simulink model "nmsRR"  (R2021a)
settings: Solver=ode15s  StartTime=0.0  StopTime=t  MaxStep=1e-2  RelTol=1e-2
StartFcn:
  | tic
StopFcn:
  | toc
  | 
  | 
  | %if GimbalLockFlag
  |  % fprintf(2, 'Almost reached Gimbal Lock of IMU. Simulation stopped.\n')
  | %end
  | 
  | %fprintf('Elapsed time: %4.2f sec (%4.2f%% realtime)\n', a, tout(end)/a*100)
undefined symbols (not defined in the file): Balance02, Balance13, BalanceTrunk, BasisStim, CompensateSwing, CompliantLeg, FlexAnkle, Ground, ICs, init_des_left, init_des_right, init_l_left, init_l_right, init_q_del, init_sensor_body, init_sensor_world, init_v_left, init_v_right, LateralControl, mParams, PreventKneeOverextension, StepDur, Target02, Target13, theta0, X, Y, Z
libraries: simulink_extras x133, nesl_utility x105, sm_lib x88, simulink x72, robotcorelib x5, dspinverses x5, dspswit3 x2, vrlib x2, robotmaniplib x1
(part 2 of 8)

== system nmsRR/Body and Contact Model/LPF 13x0.01s3 ==
  in : Inport
  Demux2 : Demux  Outputs=8
  Mux2 : Mux  Inputs=8
  Transfer Fcn (with initial outputs){,1..7} (8 alike) : simulink_extras/Additional Linear/Transfer Fcn (with initial outputs)  N=[1]  D="[0.01  1]"  Y0=0  U0=0
  Out : Outport
  wires:
  Mux2/1 -> Out/1
  in/1 -> Demux2/1
  Demux2/1 -> Transfer Fcn (with initial outputs)/1
  Transfer Fcn (with initial outputs)/1 -> Mux2/1
  Demux2/2 -> Transfer Fcn (with initial outputs)1/1
  Transfer Fcn (with initial outputs)1/1 -> Mux2/2
  Demux2/3 -> Transfer Fcn (with initial outputs)2/1
  Transfer Fcn (with initial outputs)2/1 -> Mux2/3
  Demux2/4 -> Transfer Fcn (with initial outputs)3/1
  Transfer Fcn (with initial outputs)3/1 -> Mux2/4
  Demux2/5 -> Transfer Fcn (with initial outputs)4/1
  Transfer Fcn (with initial outputs)4/1 -> Mux2/5
  Demux2/6 -> Transfer Fcn (with initial outputs)5/1
  Transfer Fcn (with initial outputs)5/1 -> Mux2/6
  Demux2/7 -> Transfer Fcn (with initial outputs)6/1
  Transfer Fcn (with initial outputs)6/1 -> Mux2/7
  Demux2/8 -> Transfer Fcn (with initial outputs)7/1
  Transfer Fcn (with initial outputs)7/1 -> Mux2/8

== system nmsRR/Body and Contact Model/LPF 13x0.01s4 ==
  in : Inport
  Demux2 : Demux  Outputs=8
  Mux2 : Mux  Inputs=8
  Transfer Fcn (with initial outputs) : simulink_extras/Additional Linear/Transfer Fcn (with initial outputs)  N=[1]  D="[0.01  1]"  Y0=init_q_del(1)  U0=init_q_del(1)
  Transfer Fcn (with initial outputs)1 : simulink_extras/Additional Linear/Transfer Fcn (with initial outputs)  N=[1]  D="[0.01  1]"  Y0=init_q_del(2)  U0=init_q_del(2)
  Transfer Fcn (with initial outputs)2 : simulink_extras/Additional Linear/Transfer Fcn (with initial outputs)  N=[1]  D="[0.01  1]"  Y0=init_q_del(3)  U0=init_q_del(3)
  Transfer Fcn (with initial outputs)3 : simulink_extras/Additional Linear/Transfer Fcn (with initial outputs)  N=[1]  D="[0.01  1]"  Y0=init_q_del(4)  U0=init_q_del(4)
  Transfer Fcn (with initial outputs)4 : simulink_extras/Additional Linear/Transfer Fcn (with initial outputs)  N=[1]  D="[0.01  1]"  Y0=init_q_del(5)  U0=init_q_del(5)
  Transfer Fcn (with initial outputs)5 : simulink_extras/Additional Linear/Transfer Fcn (with initial outputs)  N=[1]  D="[0.01  1]"  Y0=init_q_del(6)  U0=init_q_del(6)
  Transfer Fcn (with initial outputs)6 : simulink_extras/Additional Linear/Transfer Fcn (with initial outputs)  N=[1]  D="[0.01  1]"  Y0=0  U0=0
  Transfer Fcn (with initial outputs)7 : simulink_extras/Additional Linear/Transfer Fcn (with initial outputs)  N=[1]  D="[0.01  1]"  Y0=0  U0=0
  Out : Outport
  wires:
  Mux2/1 -> Out/1
  in/1 -> Demux2/1
  Demux2/1 -> Transfer Fcn (with initial outputs)/1
  Transfer Fcn (with initial outputs)/1 -> Mux2/1
  Demux2/2 -> Transfer Fcn (with initial outputs)1/1
  Transfer Fcn (with initial outputs)1/1 -> Mux2/2
  Demux2/3 -> Transfer Fcn (with initial outputs)2/1
  Transfer Fcn (with initial outputs)2/1 -> Mux2/3
  Demux2/4 -> Transfer Fcn (with initial outputs)3/1
  Transfer Fcn (with initial outputs)3/1 -> Mux2/4
  Demux2/5 -> Transfer Fcn (with initial outputs)4/1
  Transfer Fcn (with initial outputs)4/1 -> Mux2/5
  Demux2/6 -> Transfer Fcn (with initial outputs)5/1
  Transfer Fcn (with initial outputs)5/1 -> Mux2/6
  Demux2/7 -> Transfer Fcn (with initial outputs)6/1
  Transfer Fcn (with initial outputs)6/1 -> Mux2/7
  Demux2/8 -> Transfer Fcn (with initial outputs)7/1
  Transfer Fcn (with initial outputs)7/1 -> Mux2/8

== system nmsRR/Body and Contact Model/Push in x-direction ==
  Left/Right : Inport
  " Timer Phase 1" : Subsystem
  AND : Logic  AllPortsSameDT=off  OutDataTypeStr=boolean
  Compare To Constant : simulink/Logic and Bit Operations/Compare To Constant  relop===  const=10  OutDataTypeStr=boolean  ZeroCross=off
  Compare To Constant1 : simulink/Logic and Bit Operations/Compare To Constant  relop=<=  const=0.2  OutDataTypeStr=boolean
  Constant1 : Constant  Value=-135
  Constant3 : Constant  Value=0
  Counter : dspswit3/Counter  Direction=Up  CountEvent=Rising edge  CounterSize=User defined  MaxCount=255  InitialCount=0  Output=Count and Hit  HitValue=32  ResetInput=off  SamplesPerFrame=1  Ts=1  CntDtype=double  HitDtype=Logical
  External Force and Torque : sm_lib/Forces and Torques/External Force and Torque  ForceResolutionFrame=AttachedFrame  EnableForceX=on  EnableForceY=off  EnableForceZ=off  EnableForce=off  TorqueResolutionFrame=AttachedFrame  EnableTorqueX=off  EnableTorqueY=off  EnableTorqueZ=off  EnableTorque=off
  Switch : Switch  Criteria=u2 > Threshold
  Terminator2 : Terminator
  conversion : nesl_utility/Simulink-PS Converter  PhysicalDomain=network_engine_domain  SubClassName=ps_input  LeftPortType=input  RightPortType=output  PseudoPeriodic=off  Frequencies=[]  NoiseDistribution=none  NoiseParameters=[]  Unit=N  AffineConversion=off  FilteringAndDerivatives=zero  SimscapeFilterOrder=1  InputFilterTimeConstant=.001  UdotUserProvided=0
      settings: SourceProductBaseCode=PW,SS
  External Force [100 N] : PMIOPort  Side=Right
  wires:
  " Timer Phase 1"/1(Out) -> Compare To Constant1/1
  Compare To Constant/1 -> AND/1, " Timer Phase 1"/1(R)
  Counter/2 -> Terminator2/1
  Compare To Constant1/1 -> AND/2
  Left/Right/1 -> Counter/1
  Constant3/1 -> Switch/3
  AND/1 -> Switch/2
  Switch/1 -> conversion/1
  Constant1/1 -> Switch/1
  Counter/1 -> Compare To Constant/1
  connections:
  conversion/RConn1 -- External Force and Torque/LConn1
  External Force and Torque/RConn1 -- External Force [100 N]/RConn1

== system nmsRR/Body and Contact Model/Push in y-direction ==
  Left/Right : Inport
  " Timer Phase 1" : Subsystem
  AND : Logic  AllPortsSameDT=off  OutDataTypeStr=boolean
  Compare To Constant : simulink/Logic and Bit Operations/Compare To Constant  relop===  const=10  OutDataTypeStr=boolean  ZeroCross=off
  Compare To Constant1 : simulink/Logic and Bit Operations/Compare To Constant  relop=<=  const=0.2  OutDataTypeStr=boolean
  Constant1 : Constant  Value=-360
  Constant3 : Constant  Value=0
  Counter : dspswit3/Counter  Direction=Up  CountEvent=Rising edge  CounterSize=User defined  MaxCount=255  InitialCount=0  Output=Count and Hit  HitValue=32  ResetInput=off  SamplesPerFrame=1  Ts=1  CntDtype=double  HitDtype=Logical
  External Force and Torque : sm_lib/Forces and Torques/External Force and Torque  ForceResolutionFrame=AttachedFrame  EnableForceX=off  EnableForceY=off  EnableForceZ=on  EnableForce=off  TorqueResolutionFrame=AttachedFrame  EnableTorqueX=off  EnableTorqueY=off  EnableTorqueZ=off  EnableTorque=off
  Switch : Switch  Criteria=u2 > Threshold
  Terminator2 : Terminator
  conversion : nesl_utility/Simulink-PS Converter  PhysicalDomain=network_engine_domain  SubClassName=ps_input  LeftPortType=input  RightPortType=output  PseudoPeriodic=off  Frequencies=[]  NoiseDistribution=none  NoiseParameters=[]  Unit=N  AffineConversion=off  FilteringAndDerivatives=zero  SimscapeFilterOrder=1  InputFilterTimeConstant=.001  UdotUserProvided=0
      settings: SourceProductBaseCode=PW,SS
  External Force [100 N] : PMIOPort  Side=Right
  wires:
  " Timer Phase 1"/1(Out) -> Compare To Constant1/1
  Compare To Constant/1 -> AND/1, " Timer Phase 1"/1(R)
  Counter/2 -> Terminator2/1
  Compare To Constant1/1 -> AND/2
  Left/Right/1 -> Counter/1
  Constant3/1 -> Switch/3
  AND/1 -> Switch/2
  Switch/1 -> conversion/1
  Constant1/1 -> Switch/1
  Counter/1 -> Compare To Constant/1
  connections:
  conversion/RConn1 -- External Force and Torque/LConn1
  External Force and Torque/RConn1 -- External Force [100 N]/RConn1

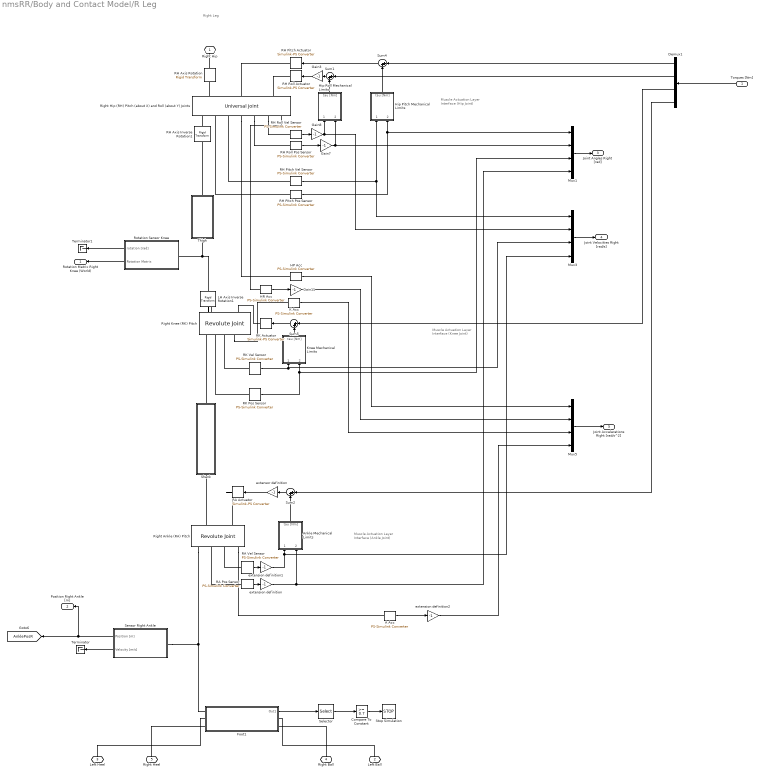
== system nmsRR/Body and Contact Model/R Leg ==
  note: Muscle Actuation
      | Layer Interface
      | (Hip Joint)
  note: Muscle Actuation
      | Layer Interface
      | (Knee Joint)
  note: Muscle Actuation
      | Layer Interface
      | (Ankle Joint)
  note: Right Leg
  Torques [Nm] : Inport
  A Acc : nesl_utility/PS-Simulink Converter  PhysicalDomain=network_engine_domain  SubClassName=ps_output  LeftPortType=input  RightPortType=output  PseudoPeriodic=off  Frequencies=[]  Unit=rad/(s^2)  AffineConversion=off
      settings: SourceProductBaseCode=PW,SS
  Ankle Mechanical Limits : Subsystem
  Compare To Constant : simulink/Logic and Bit Operations/Compare To Constant  relop=>=  const=0.7  OutDataTypeStr=boolean
  Demux1 : Demux
  Foot1 : Subsystem
  Gain{3,7..8,11} (4 alike) : Gain  Gain=-1
  HP Acc : nesl_utility/PS-Simulink Converter  PhysicalDomain=network_engine_domain  SubClassName=ps_output  LeftPortType=input  RightPortType=output  PseudoPeriodic=off  Frequencies=[]  Unit=rad/(s^2)  AffineConversion=off
      settings: SourceProductBaseCode=PW,SS
  HR Acc : nesl_utility/PS-Simulink Converter  PhysicalDomain=network_engine_domain  SubClassName=ps_output  LeftPortType=input  RightPortType=output  PseudoPeriodic=off  Frequencies=[]  Unit=rad/(s^2)  AffineConversion=off
      settings: SourceProductBaseCode=PW,SS
  Hip Pitch Mechanical Limits : Subsystem
  Hip Roll Mechanical Limits : Subsystem
  K Acc : nesl_utility/PS-Simulink Converter  PhysicalDomain=network_engine_domain  SubClassName=ps_output  LeftPortType=input  RightPortType=output  PseudoPeriodic=off  Frequencies=[]  Unit=rad/(s^2)  AffineConversion=off
      settings: SourceProductBaseCode=PW,SS
  Knee Mechanical Limits : Subsystem
  LH Axis Inverse Rotation1 : sm_lib/Frames and Transforms/Rigid Transform  TranslationMethod=None  TranslationStandardOffset=-0.5  TranslationLengthUnit=m  TranslationStandardAxis=+Y  TranslationCartesianOffset=0  TranslationROffset=0  TranslationROffsetUnits=m  TranslationZOffset=0  TranslationZOffsetUnits=m  TranslationThetaOffset=0  TranslationThetaOffsetUnits=deg  RotationMethod=RotationSequence  RotationAngleUnits=deg  RotationStandardAxis=+X  RotationAngle=-90  RotationArbitraryAxis=[0 0 1]  FollAlignAxisA=+X  BaseAlignAxisA=+Y  FollAlignAxisB=+Y  BaseAlignAxisB=+Z  RotationSequenceAxes=BaseAxes  RotationSequence=ZXZ  RotationSequenceAngles=[180 0 0]  RotationSequenceAnglesUnits=deg  RotationMatrix=[1 0 0; 0 1 0; 0 0 1]
  Mux1 : Mux
  Mux3 : Mux
  Mux5 : Mux
  RA Actuator : nesl_utility/Simulink-PS Converter  PhysicalDomain=network_engine_domain  SubClassName=ps_input  LeftPortType=input  RightPortType=output  PseudoPeriodic=off  Frequencies=[]  NoiseDistribution=none  NoiseParameters=[]  Unit=N*m  AffineConversion=off  FilteringAndDerivatives=zero  SimscapeFilterOrder=1  InputFilterTimeConstant=.001  UdotUserProvided=0
      settings: SourceProductBaseCode=PW,SS
  RA Pos Sensor : nesl_utility/PS-Simulink Converter  PhysicalDomain=network_engine_domain  SubClassName=ps_output  LeftPortType=input  RightPortType=output  PseudoPeriodic=off  Frequencies=[]  Unit=rad  AffineConversion=off
      settings: SourceProductBaseCode=PW,SS
  RA Vel Sensor : nesl_utility/PS-Simulink Converter  PhysicalDomain=network_engine_domain  SubClassName=ps_output  LeftPortType=input  RightPortType=output  PseudoPeriodic=off  Frequencies=[]  Unit=rad/s  AffineConversion=off
      settings: SourceProductBaseCode=PW,SS
  RH Pitch Pos Sensor : nesl_utility/PS-Simulink Converter  PhysicalDomain=network_engine_domain  SubClassName=ps_output  LeftPortType=input  RightPortType=output  PseudoPeriodic=off  Frequencies=[]  Unit=rad  AffineConversion=off
      settings: SourceProductBaseCode=PW,SS
  RH Pitch Vel Sensor : nesl_utility/PS-Simulink Converter  PhysicalDomain=network_engine_domain  SubClassName=ps_output  LeftPortType=input  RightPortType=output  PseudoPeriodic=off  Frequencies=[]  Unit=rad/s  AffineConversion=off
      settings: SourceProductBaseCode=PW,SS
  RH Roll Pos Sensor : nesl_utility/PS-Simulink Converter  PhysicalDomain=network_engine_domain  SubClassName=ps_output  LeftPortType=input  RightPortType=output  PseudoPeriodic=off  Frequencies=[]  Unit=rad  AffineConversion=off
      settings: SourceProductBaseCode=PW,SS
  "RH Roll Vel Sensor " : nesl_utility/PS-Simulink Converter  PhysicalDomain=network_engine_domain  SubClassName=ps_output  LeftPortType=input  RightPortType=output  PseudoPeriodic=off  Frequencies=[]  Unit=rad/s  AffineConversion=off
      settings: SourceProductBaseCode=PW,SS
  RH Axis Inverse Rotation1 : sm_lib/Frames and Transforms/Rigid Transform  TranslationMethod=None  TranslationStandardOffset=-0.5  TranslationLengthUnit=m  TranslationStandardAxis=+Y  TranslationCartesianOffset=[0 0.2 0]  TranslationROffset=0  TranslationROffsetUnits=m  TranslationZOffset=0  TranslationZOffsetUnits=m  TranslationThetaOffset=0  TranslationThetaOffsetUnits=deg  RotationMethod=RotationSequence  RotationAngleUnits=deg  RotationStandardAxis=+X  RotationAngle=-90  RotationArbitraryAxis=[0 0 1]  FollAlignAxisA=+X  BaseAlignAxisA=+Y  FollAlignAxisB=+Y  BaseAlignAxisB=+Z  RotationSequenceAxes=BaseAxes  RotationSequence=YXY  RotationSequenceAngles=[ -90 -90 0]  RotationSequenceAnglesUnits=deg  RotationMatrix=[1 0 0; 0 1 0; 0 0 1]
  RH Axis Rotation : sm_lib/Frames and Transforms/Rigid Transform  TranslationMethod=None  TranslationStandardOffset=-0  TranslationLengthUnit=m  TranslationStandardAxis=+Y  TranslationCartesianOffset=0  TranslationROffset=0  TranslationROffsetUnits=m  TranslationZOffset=0  TranslationZOffsetUnits=m  TranslationThetaOffset=0  TranslationThetaOffsetUnits=deg  RotationMethod=RotationSequence  RotationAngleUnits=deg  RotationStandardAxis=+X  RotationAngle=90  RotationArbitraryAxis=[0 0 1]  FollAlignAxisA=+X  BaseAlignAxisA=+Y  FollAlignAxisB=+Y  BaseAlignAxisB=+Z  RotationSequenceAxes=FollowerAxes  RotationSequence=XZX  RotationSequenceAngles=[-90 90 0]  RotationSequenceAnglesUnits=deg  RotationMatrix=[1 0 0; 0 1 0; 0 0 1]
  RH Pitch Actuator : nesl_utility/Simulink-PS Converter  PhysicalDomain=network_engine_domain  SubClassName=ps_input  LeftPortType=input  RightPortType=output  PseudoPeriodic=off  Frequencies=[]  NoiseDistribution=none  NoiseParameters=[]  Unit=N*m  AffineConversion=off  FilteringAndDerivatives=zero  SimscapeFilterOrder=1  InputFilterTimeConstant=.001  UdotUserProvided=0
      settings: SourceProductBaseCode=PW,SS
  RH Roll Actuator : nesl_utility/Simulink-PS Converter  PhysicalDomain=network_engine_domain  SubClassName=ps_input  LeftPortType=input  RightPortType=output  PseudoPeriodic=off  Frequencies=[]  NoiseDistribution=none  NoiseParameters=[]  Unit=N*m  AffineConversion=off  FilteringAndDerivatives=zero  SimscapeFilterOrder=1  InputFilterTimeConstant=.001  UdotUserProvided=0
      settings: SourceProductBaseCode=PW,SS
  RK Actuator : nesl_utility/Simulink-PS Converter  PhysicalDomain=network_engine_domain  SubClassName=ps_input  LeftPortType=input  RightPortType=output  PseudoPeriodic=off  Frequencies=[]  NoiseDistribution=none  NoiseParameters=[]  Unit=N*m  AffineConversion=off  FilteringAndDerivatives=zero  SimscapeFilterOrder=1  InputFilterTimeConstant=.001  UdotUserProvided=0
      settings: SourceProductBaseCode=PW,SS
  RK Pos Sensor : nesl_utility/PS-Simulink Converter  PhysicalDomain=network_engine_domain  SubClassName=ps_output  LeftPortType=input  RightPortType=output  PseudoPeriodic=off  Frequencies=[]  Unit=rad  AffineConversion=off
      settings: SourceProductBaseCode=PW,SS
  RK Vel Sensor : nesl_utility/PS-Simulink Converter  PhysicalDomain=network_engine_domain  SubClassName=ps_output  LeftPortType=input  RightPortType=output  PseudoPeriodic=off  Frequencies=[]  Unit=rad/s  AffineConversion=off
      settings: SourceProductBaseCode=PW,SS
  Right Ankle (RA) Pitch : sm_lib/Joints/Revolute Joint  JointMode=Normal  SenseConstraintForce=off  SenseConstraintForceX=off  SenseConstraintForceY=off  SenseConstraintForceZ=off  SenseConstraintTorque=off  SenseConstraintTorqueX=off  SenseConstraintTorqueY=off  SenseConstraintTorqueZ=off  SenseTotalForce=off  SenseTotalForceX=off  SenseTotalForceY=off  SenseTotalForceZ=off  SenseTotalTorque=off  SenseTotalTorqueX=off  SenseTotalTorqueY=off  SenseTotalTorqueZ=off  CompositeWrenchDir=FollowerOnBase  CompositeWrenchFrame=FollowerFrame  EquilibriumPosition=0  EquilibriumPositionUnits=deg  SpringStiffness=0  SpringStiffnessUnits=N*m/deg  DampingCoefficient=0  DampingCoefficientUnits=N*m/(deg/s)  TorqueActuationMode=InputTorque  MotionActuationMode=ComputedMotion  SensePosition=on  SenseVelocity=on  SenseAcceleration=on  SenseTorqueForce=off  SenseLowerLimitTorqueForce=off  SenseUpperLimitTorqueForce=off  LowerLimitSpecify=off  LowerLimitBound=-90  LowerLimitBoundUnits=deg  LowerLimitStiffness=1e4  LowerLimitStiffnessUnits=N*m/deg  LowerLimitDamping=10  LowerLimitDampingUnits=N*m/(deg/s)  LowerLimitTransitionRegionWidth=0.1  LowerLimitTransitionRegionWidthUnits=deg  UpperLimitSpecify=off  UpperLimitBound=90  UpperLimitBoundUnits=deg  UpperLimitStiffness=1e4  UpperLimitStiffnessUnits=N*m/deg  UpperLimitDamping=10  UpperLimitDampingUnits=N*m/(deg/s)  UpperLimitTransitionRegionWidth=0.1  UpperLimitTransitionRegionWidthUnits=deg  PositionTargetSpecify=on  PositionTargetPriority=High  PositionTargetValue=-ICs.rLeg.ankle.qP0  PositionTargetValueUnits=rad  VelocityTargetSpecify=on  VelocityTargetPriority=High  VelocityTargetValue=0  VelocityTargetValueUnits=rad/s
  Right Hip (RH) Pitch (about X) and Roll (about Y) Joints : sm_lib/Joints/Universal Joint  JointMode=Normal  SenseConstraintForce=off  SenseConstraintForceX=off  SenseConstraintForceY=off  SenseConstraintForceZ=off  SenseConstraintTorque=off  SenseConstraintTorqueX=off  SenseConstraintTorqueY=off  SenseConstraintTorqueZ=off  SenseTotalForce=off  SenseTotalForceX=off  SenseTotalForceY=off  SenseTotalForceZ=off  SenseTotalTorque=off  SenseTotalTorqueX=off  SenseTotalTorqueY=off  SenseTotalTorqueZ=off  CompositeWrenchDir=FollowerOnBase  CompositeWrenchFrame=FollowerFrame  RxEquilibriumPosition=0  RxEquilibriumPositionUnits=deg  RxSpringStiffness=0  RxSpringStiffnessUnits=N*m/deg  RxDampingCoefficient=0  RxDampingCoefficientUnits=N*m/(deg/s)  RxTorqueActuationMode=InputTorque  RxMotionActuationMode=ComputedMotion  RxSensePosition=on  RxSenseVelocity=on  RxSenseAcceleration=on  RxSenseTorqueForce=off  RxSenseLowerLimitTorqueForce=off  RxSenseUpperLimitTorqueForce=off  RxLowerLimitSpecify=off  RxLowerLimitBound=-90  RxLowerLimitBoundUnits=deg  RxLowerLimitStiffness=1e4  RxLowerLimitStiffnessUnits=N*m/deg  RxLowerLimitDamping=10  RxLowerLimitDampingUnits=N*m/(deg/s)  RxLowerLimitTransitionRegionWidth=0.1  RxLowerLimitTransitionRegionWidthUnits=deg  RxUpperLimitSpecify=off  RxUpperLimitBound=90  RxUpperLimitBoundUnits=deg  RxUpperLimitStiffness=1e4  RxUpperLimitStiffnessUnits=N*m/deg  RxUpperLimitDamping=10  RxUpperLimitDampingUnits=N*m/(deg/s)  RxUpperLimitTransitionRegionWidth=0.1  RxUpperLimitTransitionRegionWidthUnits=deg  RxPositionTargetSpecify=on  RxPositionTargetPriority=High  RxPositionTargetValue=ICs.rLeg.hip.qP0  RxPositionTargetValueUnits=rad  RxVelocityTargetSpecify=on  RxVelocityTargetPriority=High  RxVelocityTargetValue=0  RxVelocityTargetValueUnits=rad/s  RyEquilibriumPosition=0  RyEquilibriumPositionUnits=deg  RySpringStiffness=0  RySpringStiffnessUnits=N*m/deg  RyDampingCoefficient=0  RyDampingCoefficientUnits=N*m/(deg/s)  RyTorqueActuationMode=InputTorque  RyMotionActuationMode=ComputedMotion  RySensePosition=on  RySenseVelocity=on  RySenseAcceleration=on  RySenseTorqueForce=off  RySenseLowerLimitTorqueForce=off  RySenseUpperLimitTorqueForce=off  RyLowerLimitSpecify=off  RyLowerLimitBound=-90  RyLowerLimitBoundUnits=deg  RyLowerLimitStiffness=1e4  RyLowerLimitStiffnessUnits=N*m/deg  RyLowerLimitDamping=10  RyLowerLimitDampingUnits=N*m/(deg/s)  RyLowerLimitTransitionRegionWidth=0.1  RyLowerLimitTransitionRegionWidthUnits=deg  RyUpperLimitSpecify=off  RyUpperLimitBound=90  RyUpperLimitBoundUnits=deg  RyUpperLimitStiffness=1e4  RyUpperLimitStiffnessUnits=N*m/deg  RyUpperLimitDamping=10  RyUpperLimitDampingUnits=N*m/(deg/s)  RyUpperLimitTransitionRegionWidth=0.1  RyUpperLimitTransitionRegionWidthUnits=deg  RyPositionTargetSpecify=on  RyPositionTargetPriority=High  RyPositionTargetValue=-ICs.rLeg.hip.qR0  RyPositionTargetValueUnits=rad  RyVelocityTargetSpecify=on  RyVelocityTargetPriority=High  RyVelocityTargetValue=0  RyVelocityTargetValueUnits=rad/s
  Right Knee (RK) Pitch : sm_lib/Joints/Revolute Joint  JointMode=Normal  SenseConstraintForce=off  SenseConstraintForceX=off  SenseConstraintForceY=off  SenseConstraintForceZ=off  SenseConstraintTorque=off  SenseConstraintTorqueX=off  SenseConstraintTorqueY=off  SenseConstraintTorqueZ=off  SenseTotalForce=off  SenseTotalForceX=off  SenseTotalForceY=off  SenseTotalForceZ=off  SenseTotalTorque=off  SenseTotalTorqueX=off  SenseTotalTorqueY=off  SenseTotalTorqueZ=off  CompositeWrenchDir=FollowerOnBase  CompositeWrenchFrame=FollowerFrame  EquilibriumPosition=0  EquilibriumPositionUnits=deg  SpringStiffness=0  SpringStiffnessUnits=N*m/deg  DampingCoefficient=0  DampingCoefficientUnits=N*m/(deg/s)  TorqueActuationMode=InputTorque  MotionActuationMode=ComputedMotion  SensePosition=on  SenseVelocity=on  SenseAcceleration=on  SenseTorqueForce=on  SenseLowerLimitTorqueForce=off  SenseUpperLimitTorqueForce=off  LowerLimitSpecify=off  LowerLimitBound=-90  LowerLimitBoundUnits=deg  LowerLimitStiffness=1e4  LowerLimitStiffnessUnits=N*m/deg  LowerLimitDamping=10  LowerLimitDampingUnits=N*m/(deg/s)  LowerLimitTransitionRegionWidth=0.1  LowerLimitTransitionRegionWidthUnits=deg  UpperLimitSpecify=off  UpperLimitBound=90  UpperLimitBoundUnits=deg  UpperLimitStiffness=1e4  UpperLimitStiffnessUnits=N*m/deg  UpperLimitDamping=10  UpperLimitDampingUnits=N*m/(deg/s)  UpperLimitTransitionRegionWidth=0.1  UpperLimitTransitionRegionWidthUnits=deg  PositionTargetSpecify=on  PositionTargetPriority=High  PositionTargetValue=ICs.rLeg.knee.qP0  PositionTargetValueUnits=rad  VelocityTargetSpecify=on  VelocityTargetPriority=High  VelocityTargetValue=0  VelocityTargetValueUnits=rad/s
  Rotation Sensor Knee : Subsystem
  Selector : Selector  InputPortWidth=3  IndexOptions=Index vector (dialog)  Indices=[2]  OutputSizes=1
  Sensor Right Ankle : Subsystem
  Shank : Subsystem
  Stop Simulation : Stop
  Sum{1..2,4..5} (4 alike) : Sum  Inputs=|++
  Terminator : Terminator
  Terminator1 : Terminator
  Thigh : Subsystem
  extension definition : Gain  Gain=-1
  extension definition1 : Gain  Gain=-1
  extension definition2 : Gain  Gain=-1
  extensor definition : Gain  Gain=-1
  Right Hip : PMIOPort  Side=Left
  "Left Ball " : PMIOPort  Port=2  Side=Right
  Left Heel : PMIOPort  Port=3  Side=Right
  Right Ball : PMIOPort  Port=4  Side=Right
  Right Heel : PMIOPort  Port=5  Side=Right
  Rotation Matrix Right Knee (World) : Outport
  Position Right Ankle [m] : Outport  Port=2
  Joint Angles Right [rad] : Outport  Port=3
  "Joint Velocities Right [rad/s] " : Outport  Port=4
  Joint Accelerations Right [rad/s^2] : Outport  Port=5
  tag scope: AnklePosR=global
  wires:
  Hip Pitch Mechanical Limits/1(tau [Nm]) -> Sum4/2
  RH Pitch Vel Sensor/1 -> Mux3/1, Hip Pitch Mechanical Limits/1(dq [rad/s])
  Hip Roll Mechanical Limits/1(tau [Nm]) -> Sum1/2
  RK Pos Sensor/1 -> Knee Mechanical Limits/2(q [rad]), Mux1/3
  Demux1/3 -> Sum5/1
  RK Vel Sensor/1 -> Mux3/3, Knee Mechanical Limits/1(dq [rad/s])
  RH Pitch Pos Sensor/1 -> Hip Pitch Mechanical Limits/2(q [rad]), Mux1/1
  RH Roll Pos Sensor/1 -> Gain7/1
  Demux1/1 -> Sum4/1
  Sum2/1 -> extensor definition/1
  RA Vel Sensor/1 -> extension definition1/1
  Demux1/4 -> Sum2/1
  Ankle Mechanical Limits/1(tau [Nm]) -> Sum2/2
  RA Pos Sensor/1 -> extension definition/1
  extension definition/1 -> Mux1/4, Ankle Mechanical Limits/2(q [rad])
  extension definition1/1 -> Mux3/4, Ankle Mechanical Limits/1(dq [rad/s])
  Sum4/1 -> RH Pitch Actuator/1
  Sum1/1 -> Gain3/1
  Gain3/1 -> RH Roll Actuator/1
  Sum5/1 -> RK Actuator/1
  extensor definition/1 -> RA Actuator/1
  "RH Roll Vel Sensor "/1 -> Gain8/1
  Gain8/1 -> Mux3/2, Hip Roll Mechanical Limits/1(dq [rad/s])
  Gain7/1 -> Mux1/2, Hip Roll Mechanical Limits/2(q [rad])
  Demux1/2 -> Sum1/1
  Mux3/1 -> "Joint Velocities Right [rad/s] "/1
  Mux5/1 -> Joint Accelerations Right [rad/s^2]/1
  HP Acc/1 -> Mux5/1
  HR Acc/1 -> Gain11/1
  Gain11/1 -> Mux5/2
  K Acc/1 -> Mux5/3
  A Acc/1 -> extension definition2/1
  extension definition2/1 -> Mux5/4
  Knee Mechanical Limits/1(tau [Nm]) -> Sum5/2
  Rotation Sensor Knee/1(rotation [rad]) -> Terminator1/1
  Sensor Right Ankle/1(Position [m]) -> Position Right Ankle [m]/1, [AnklePosR]
  Rotation Sensor Knee/2(Rotation Matrix) -> Rotation Matrix Right Knee (World)/1
  Selector/1 -> Compare To Constant/1
  Compare To Constant/1 -> Stop Simulation/1
  Foot1/1(Out1) -> Selector/1
  Sensor Right Ankle/2(Velocity [m/s]) -> Terminator/1
  Torques [Nm]/1 -> Demux1/1
  Mux1/1 -> Joint Angles Right [rad]/1
  connections:
  RH Axis Rotation/LConn1 -- Right Hip/RConn1
  RK Vel Sensor/LConn1 -- Right Knee (RK) Pitch/RConn3
  RK Pos Sensor/LConn1 -- Right Knee (RK) Pitch/RConn2
  RH Pitch Pos Sensor/LConn1 -- Right Hip (RH) Pitch (about X) and Roll (about Y) Joints/RConn2
  RH Pitch Vel Sensor/LConn1 -- Right Hip (RH) Pitch (about X) and Roll (about Y) Joints/RConn3
  Right Hip (RH) Pitch (about X) and Roll (about Y) Joints/LConn1 -- RH Axis Rotation/RConn1
  Shank/LConn1 -- Right Knee (RK) Pitch/RConn1
  LH Axis Inverse Rotation1/RConn1 -- Right Knee (RK) Pitch/LConn1
  Right Ankle (RA) Pitch/LConn1 -- Shank/RConn1
  RA Vel Sensor/LConn1 -- Right Ankle (RA) Pitch/RConn3
  RA Pos Sensor/LConn1 -- Right Ankle (RA) Pitch/RConn2
  RH Axis Inverse Rotation1/LConn1 -- Right Hip (RH) Pitch (about X) and Roll (about Y) Joints/RConn1
  Right Hip (RH) Pitch (about X) and Roll (about Y) Joints/RConn5 -- RH Roll Pos Sensor/LConn1
  Right Hip (RH) Pitch (about X) and Roll (about Y) Joints/RConn6 -- "RH Roll Vel Sensor "/LConn1
  Right Hip (RH) Pitch (about X) and Roll (about Y) Joints/RConn4 -- HP Acc/LConn1
  Right Hip (RH) Pitch (about X) and Roll (about Y) Joints/RConn7 -- HR Acc/LConn1
  Right Knee (RK) Pitch/RConn4 -- K Acc/LConn1
  Right Ankle (RA) Pitch/RConn4 -- A Acc/LConn1
  Right Heel/RConn1 -- Foot1/LConn3
  Left Heel/RConn1 -- Foot1/LConn2
  Right Ball/RConn1 -- Foot1/RConn2
  "Left Ball "/RConn1 -- Foot1/RConn1
  Thigh/LConn1 -- RH Axis Inverse Rotation1/RConn1
  Thigh/RConn1 -- LH Axis Inverse Rotation1/LConn1 -- Rotation Sensor Knee/LConn1
  Right Ankle (RA) Pitch/RConn1 -- Sensor Right Ankle/LConn1 -- Foot1/LConn1
  RK Actuator/RConn1 -- Right Knee (RK) Pitch/LConn2
  RA Actuator/RConn1 -- Right Ankle (RA) Pitch/LConn2
  RH Pitch Actuator/RConn1 -- Right Hip (RH) Pitch (about X) and Roll (about Y) Joints/LConn2
  RH Roll Actuator/RConn1 -- Right Hip (RH) Pitch (about X) and Roll (about Y) Joints/LConn3

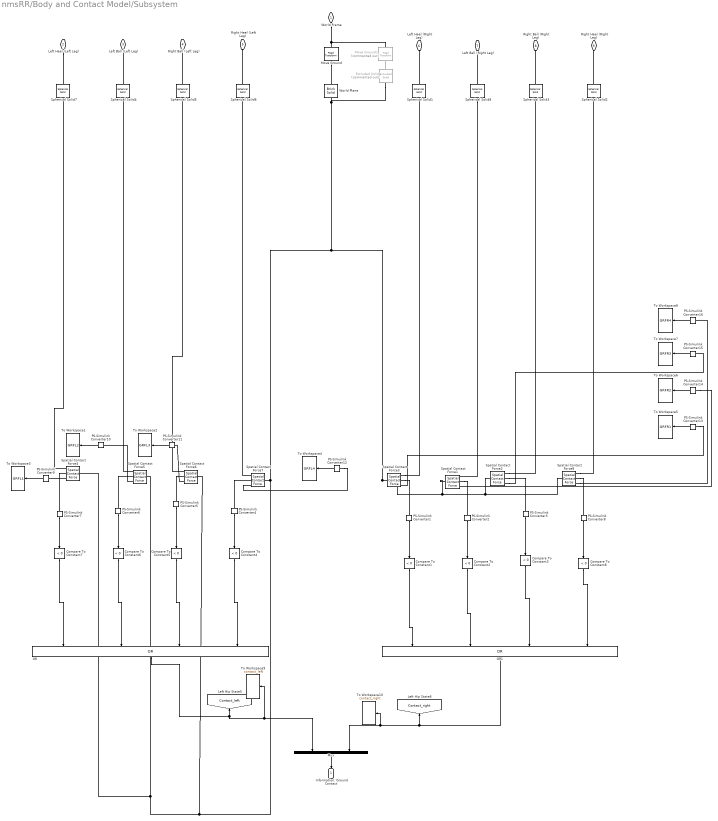
== system nmsRR/Body and Contact Model/Subsystem ==
  Compare To Constant{1..8} (8 alike) : simulink/Logic and Bit Operations/Compare To Constant  relop=<  const=0  OutDataTypeStr=boolean
  Extruded Solid : sm_lib/Body Elements/Extruded Solid  Commented=on  GraphicAmbientColor=[0.15 0.15 0.15 1.0]  BasedOnType=Density  CenterOfMass=[0 0 0]  CenterOfMassUnits=m  GraphicDiffuseColor=[0.5 0.5 0.5]  ExportConvexHullGeometry=on  ExtrusionCrossSection=[Ground]  ExtrusionCrossSectionUnits=m  Density=1000  DensityUnits=kg/m^3  DoExposeReferenceFrame=on  GraphicEmissiveColor=[0.0 0.0 0.0 1.0]  ExportEntireGeometry=off  ExtrusionLength=10  ExtrusionLengthUnits=m  ExtrusionType=General  SerializedFrames=<Frames/>  MarkerShape=Sphere  MarkerSize=10  GraphicType=FromGeometry  InertiaType=CalculateFromGeometry  Mass=1  MassUnits=kg  MomentsOfInertia=[1 1 1]  MomentsOfInertiaUnits=kg*m^2  PolygonNumSides=3  GraphicOpacity=1.0  PolygonOuterRadius=1  PolygonOuterRadiusUnits=m  ProductsOfInertia=[0 0 0]  ProductsOfInertiaUnits=kg*m^2  GraphicShininess=75  GraphicSpecularColor=[0.5 0.5 0.5 1.0]  GraphicVisPropType=SimpleVisualProperties
  Move Ground : sm_lib/Frames and Transforms/Rigid Transform  TranslationMethod=StandardAxis  TranslationStandardOffset=-0.05  TranslationLengthUnit=m  TranslationStandardAxis=+Y  TranslationCartesianOffset=0  TranslationROffset=0  TranslationROffsetUnits=m  TranslationZOffset=0  TranslationZOffsetUnits=m  TranslationThetaOffset=0  TranslationThetaOffsetUnits=deg  RotationMethod=None  RotationAngleUnits=deg  RotationStandardAxis=+X  RotationAngle=-90  RotationArbitraryAxis=[0 0 1]  FollAlignAxisA=+X  BaseAlignAxisA=+Y  FollAlignAxisB=+Y  BaseAlignAxisB=+Z  RotationSequenceAxes=BaseAxes  RotationSequence=ZXZ  RotationSequenceAngles=[180 0 0]  RotationSequenceAnglesUnits=deg  RotationMatrix=[1 0 0; 0 1 0; 0 0 1]
  Move Ground1 : sm_lib/Frames and Transforms/Rigid Transform  Commented=on  TranslationMethod=StandardAxis  TranslationStandardOffset=-0.2  TranslationLengthUnit=m  TranslationStandardAxis=+X  TranslationCartesianOffset=0  TranslationROffset=0  TranslationROffsetUnits=m  TranslationZOffset=0  TranslationZOffsetUnits=m  TranslationThetaOffset=0  TranslationThetaOffsetUnits=deg  RotationMethod=RotationSequence  RotationAngleUnits=deg  RotationStandardAxis=+X  RotationAngle=-90  RotationArbitraryAxis=[0 0 1]  FollAlignAxisA=+X  BaseAlignAxisA=+Y  FollAlignAxisB=+Y  BaseAlignAxisB=+Z  RotationSequenceAxes=BaseAxes  RotationSequence=YZX  RotationSequenceAngles=[180 -90 0]  RotationSequenceAnglesUnits=deg  RotationMatrix=[1 0 0; 0 1 0; 0 0 1]
  Mux : Mux  Inputs=2
  OR : Logic  Operator=OR  Inputs=4  AllPortsSameDT=off  OutDataTypeStr=boolean
  OR1 : Logic  Operator=OR  Inputs=4  AllPortsSameDT=off  OutDataTypeStr=boolean
  PS-Simulink Converter{1..8} (8 alike) : nesl_utility/PS-Simulink Converter  PhysicalDomain=network_engine_domain  SubClassName=ps_output  LeftPortType=input  RightPortType=output  PseudoPeriodic=off  Frequencies=[]  Unit=m  AffineConversion=off
      settings: SourceProductBaseCode=PW,SS
  PS-Simulink Converter{9..16} (8 alike) : nesl_utility/PS-Simulink Converter  PhysicalDomain=network_engine_domain  SubClassName=ps_output  LeftPortType=input  RightPortType=output  PseudoPeriodic=off  Frequencies=[]  Unit=N  AffineConversion=off
      settings: SourceProductBaseCode=PW,SS
  Spatial Contact Force{1..8} (8 alike) : sm_lib/Forces and Torques/Spatial Contact Force  CoefficientOfDynamicFriction=mParams.Contacts.mu_k  CoefficientOfStaticFriction=mParams.Contacts.mu_s  SenseContactBaseRotation=off  SenseContactBaseTranslation=off  NormalDamping=mParams.Contacts.damping  NormalDampingUnits=N/(m/s)  SenseContactFollowerRotation=off  SenseContactFollowerTranslation=off  SenseContactSignal=off  NormalStiffness=mParams.Contacts.stiffness  NormalStiffnessUnits=N/m  FrictionalCriticalVelocity=mParams.Contacts.vLimit  FrictionalCriticalVelocityUnits=m/s  ZeroCrossDetectContactStartAndEnd=off  FrictionType=SmoothStickSlip  SenseFrictionalForceMagnitude=off  SenseNormalForceMagnitude=on  NormalForceType=SmoothSpringDamper  SenseNormalVelocity=off  SenseSeparationDistance=on  SenseTangentialVelocity=off  SenseTangentialVelocityMagnitude=off  NormalTransitionRegionWidth=mParams.Contacts.depths  NormalTransitionRegionWidthUnits=m
  Spherical Solid{1..8} (8 alike) : sm_lib/Body Elements/Spherical Solid  GraphicAmbientColor=[0.15 0.15 0.15 1.0]  BasedOnType=Mass  CenterOfMass=[0 0 0]  CenterOfMassUnits=m  GraphicDiffuseColor=[0.5 0.5 0.5]  Density=1000  DensityUnits=kg/m^3  DoExposeReferenceFrame=on  GraphicEmissiveColor=[0.0 0.0 0.0 1.0]  ExportEntireGeometry=on  SerializedExposedGeometries=<ExposedGeometries><ExposedGeometry><RawGeometryId>entire</RawGeometryId><ExposedGeometryId>G</ExposedGeometryId></ExposedGeometry></ExposedGeometries>  SerializedFrames=<Frames/>  MarkerShape=Sphere  MarkerSize=10  GraphicType=FromGeometry  InertiaType=CalculateFromGeometry  Mass=1  MassUnits=g  MomentsOfInertia=[1 1 1]  MomentsOfInertiaUnits=kg*m^2  GraphicOpacity=1.0  ProductsOfInertia=[0 0 0]  ProductsOfInertiaUnits=kg*m^2  GraphicShininess=75  GraphicSpecularColor=[0.5 0.5 0.5 1.0]  SphereRadius=mParams.Contacts.size  SphereRadiusUnits=m  GraphicVisPropType=SimpleVisualProperties
  To Workspace1 : ToWorkspace  VariableName=GRFL2  SampleTime=-1
      settings: Save2DSignal=2-D array (concatenate along first dimension)
  To Workspace10 : ToWorkspace  VariableName=contact_right  SampleTime=-1
      settings: Save2DSignal=2-D array (concatenate along first dimension)
  To Workspace2 : ToWorkspace  VariableName=GRFL3  SampleTime=-1
      settings: Save2DSignal=2-D array (concatenate along first dimension)
  To Workspace3 : ToWorkspace  VariableName=GRFL1  SampleTime=-1
      settings: Save2DSignal=2-D array (concatenate along first dimension)
  To Workspace4 : ToWorkspace  VariableName=GRFL4  SampleTime=-1
      settings: Save2DSignal=2-D array (concatenate along first dimension)
  To Workspace5 : ToWorkspace  VariableName=GRFR1  SampleTime=-1
      settings: Save2DSignal=2-D array (concatenate along first dimension)
  To Workspace6 : ToWorkspace  VariableName=GRFR2  SampleTime=-1
      settings: Save2DSignal=2-D array (concatenate along first dimension)
  To Workspace7 : ToWorkspace  VariableName=GRFR3  SampleTime=-1
      settings: Save2DSignal=2-D array (concatenate along first dimension)
  To Workspace8 : ToWorkspace  VariableName=GRFR4  SampleTime=-1
      settings: Save2DSignal=2-D array (concatenate along first dimension)
  To Workspace9 : ToWorkspace  VariableName=contact_left  SampleTime=-1
      settings: Save2DSignal=2-D array (concatenate along first dimension)
  World Plane : sm_lib/Body Elements/Brick Solid  GraphicAmbientColor=[0.15 0.15 0.15 1.0]  BasedOnType=Density  BrickDimensions=[400 0.1 400]  BrickDimensionUnits=m  CenterOfMass=[0 0 0]  CenterOfMassUnits=m  GraphicDiffuseColor=[1.0 1.0 0.8]  Density=1000  DensityUnits=kg/(m^3)  DoExposeReferenceFrame=on  GraphicEmissiveColor=[0.0 0.0 0.0 1.0]  ExportEntireGeometry=on  SerializedFrames=<Frames/>  MarkerShape=Sphere  MarkerSize=10  GraphicType=FromGeometry  InertiaType=CalculateFromGeometry  Mass=1  MassUnits=kg  MomentsOfInertia=[1 1 1]  MomentsOfInertiaUnits=kg*m^2  GraphicOpacity=0.5  ProductsOfInertia=[0 0 0]  ProductsOfInertiaUnits=kg*m^2  GraphicShininess=75  GraphicSpecularColor=[0.5 0.5 0.5 1.0]  GraphicVisPropType=SimpleVisualProperties
  World Frame : PMIOPort  Side=Left
  Left Heel (Left Leg) : PMIOPort  Port=2  Side=Right
  Left Ball (Left Leg) : PMIOPort  Port=3  Side=Right
  Right Ball (Left Leg) : PMIOPort  Port=4  Side=Right
  Right Heel (Left Leg) : PMIOPort  Port=5  Side=Right
  Left Heel (Right Leg) : PMIOPort  Port=6  Side=Right
  Left Ball (Right Leg) : PMIOPort  Port=7  Side=Right
  Right Ball (Right Leg) : PMIOPort  Port=8  Side=Right
  Right Heel (Right Leg) : PMIOPort  Port=9  Side=Right
  Information: Ground Contact : Outport
  tag scope: Contact_left=global, Contact_right=global
  wires:
  Compare To Constant1/1 -> OR1/1
  PS-Simulink Converter4/1 -> Compare To Constant4/1
  PS-Simulink Converter5/1 -> Compare To Constant5/1
  Compare To Constant4/1 -> OR/4
  PS-Simulink Converter3/1 -> Compare To Constant3/1
  Compare To Constant6/1 -> OR/2
  PS-Simulink Converter1/1 -> Compare To Constant1/1
  PS-Simulink Converter8/1 -> Compare To Constant8/1
  Compare To Constant3/1 -> OR1/3
  Compare To Constant8/1 -> OR1/4
  PS-Simulink Converter6/1 -> Compare To Constant6/1
  PS-Simulink Converter7/1 -> Compare To Constant7/1
  Compare To Constant2/1 -> OR1/2
  Compare To Constant5/1 -> OR/3
  Compare To Constant7/1 -> OR/1
  PS-Simulink Converter2/1 -> Compare To Constant2/1
  OR1/1 -> To Workspace10/1, Mux/2, [Contact_right]
  Mux/1 -> Information: Ground Contact/1
  OR/1 -> To Workspace9/1, Mux/1, [Contact_left]
  PS-Simulink Converter9/1 -> To Workspace3/1
  PS-Simulink Converter10/1 -> To Workspace1/1
  PS-Simulink Converter11/1 -> To Workspace2/1
  PS-Simulink Converter12/1 -> To Workspace4/1
  PS-Simulink Converter13/1 -> To Workspace5/1
  PS-Simulink Converter14/1 -> To Workspace6/1
  PS-Simulink Converter15/1 -> To Workspace7/1
  PS-Simulink Converter16/1 -> To Workspace8/1
  connections:
  Spatial Contact Force7/RConn1 -- Spherical Solid6/LConn1
  Spatial Contact Force5/RConn2 -- PS-Simulink Converter6/LConn1
  Spatial Contact Force7/RConn2 -- PS-Simulink Converter4/LConn1
  Spherical Solid5/RConn1 -- Right Ball (Left Leg)/RConn1
  Spherical Solid8/LConn1 -- Spatial Contact Force1/RConn1
  Spatial Contact Force6/RConn1 -- Spherical Solid5/LConn1
  Spatial Contact Force3/RConn2 -- PS-Simulink Converter1/LConn1
  Spatial Contact Force5/RConn1 -- Spherical Solid4/LConn1
  Spatial Contact Force6/RConn2 -- PS-Simulink Converter5/LConn1
  Spatial Contact Force2/RConn1 -- Spherical Solid3/LConn1
  Spatial Contact Force3/RConn1 -- Spherical Solid1/LConn1
  Spherical Solid6/RConn1 -- Right Heel (Left Leg)/RConn1
  Spatial Contact Force4/RConn2 -- PS-Simulink Converter7/LConn1
  Spatial Contact Force4/RConn1 -- Spherical Solid7/LConn1
  Spherical Solid4/RConn1 -- Left Ball (Left Leg)/RConn1
  Spatial Contact Force8/RConn1 -- Spherical Solid2/LConn1
  Left Heel (Left Leg)/RConn1 -- Spherical Solid7/RConn1
  Spherical Solid2/RConn1 -- Right Heel (Right Leg)/RConn1
  Spherical Solid1/RConn1 -- Left Heel (Right Leg)/RConn1
  Spherical Solid3/RConn1 -- Right Ball (Right Leg)/RConn1
  Spherical Solid8/RConn1 -- Left Ball (Right Leg)/RConn1
  Spatial Contact Force2/RConn2 -- PS-Simulink Converter3/LConn1
  Spatial Contact Force8/RConn2 -- PS-Simulink Converter8/LConn1
  Spatial Contact Force1/RConn2 -- PS-Simulink Converter2/LConn1
  Spatial Contact Force6/LConn1 -- Extruded Solid/LConn1 -- World Plane/LConn1 -- Spatial Contact Force1/LConn1 -- Spatial Contact Force8/LConn1 -- Spatial Contact Force2/LConn1 -- Spatial Contact Force3/LConn1 -- Spatial Contact Force7/LConn1 -- Spatial Contact Force4/LConn1 -- Spatial Contact Force5/LConn1
  Extruded Solid/RConn1 -- Move Ground1/RConn1
  World Frame/RConn1 -- Move Ground1/LConn1 -- Move Ground/LConn1
  Move Ground/RConn1 -- World Plane/RConn1
  Spatial Contact Force4/RConn3 -- PS-Simulink Converter9/LConn1
  Spatial Contact Force5/RConn3 -- PS-Simulink Converter10/LConn1
  Spatial Contact Force6/RConn3 -- PS-Simulink Converter11/LConn1
  PS-Simulink Converter12/LConn1 -- Spatial Contact Force7/RConn3
  PS-Simulink Converter13/LConn1 -- Spatial Contact Force3/RConn3
  PS-Simulink Converter14/LConn1 -- Spatial Contact Force1/RConn3
  Spatial Contact Force2/RConn3 -- PS-Simulink Converter15/LConn1
  Spatial Contact Force8/RConn3 -- PS-Simulink Converter16/LConn1

== system nmsRR/Body and Contact Model/Trunk (floating base) ==
  Solid : sm_lib/Body Elements/Brick Solid  GraphicAmbientColor=[0.15 0.15 0.15 1.0]  BasedOnType=Density  BrickDimensions=[mParams.bodies.trunk.d mParams.bodies.trunk.l mParams.bodies.trunk.b]  BrickDimensionUnits=m  CenterOfMass=mParams.bodies.trunk.CG  CenterOfMassUnits=m  GraphicDiffuseColor=[0.5 1 0.5]  Density=2.7  DensityUnits=g/cm^3  DoExposeReferenceFrame=on  GraphicEmissiveColor=[0 0 0 1.0]  ExportEntireGeometry=off  SerializedFrames=<Frames><Frame><Id>Frame1</Id><Value><Name>CG</Name><Origin><Source>CenterOfMassFrame</Source><FeatureName></FeatureName></Origin><PrimaryAxis><DefinedDirection>+Z</DefinedDirection><Source>ReferenceFrame</Source><SourceDirection>+Z</SourceDirection><FeatureName></FeatureName></PrimaryAxis><SecondaryAxis><DefinedDirection>+X</DefinedDirection><Source>ReferenceFrame</Source><SourceDirection>+X</SourceDirection><FeatureName></FeatureName></SecondaryAxis></Value></Frame></Frames>  MarkerShape=Cube  MarkerSize=100  GraphicType=FromGeometry  InertiaType=Custom  Mass=mParams.bodies.trunk.m  MassUnits=kg  MomentsOfInertia=mParams.bodies.trunk.In  MomentsOfInertiaUnits=kg*m^2  GraphicOpacity=0.5  ProductsOfInertia=[0 0 0]  ProductsOfInertiaUnits=kg*m^2  GraphicShininess=75  GraphicSpecularColor=[0.5 0.5 0.5 1.0]  GraphicVisPropType=SimpleVisualProperties
  Transform CG to LH : sm_lib/Frames and Transforms/Rigid Transform  TranslationMethod=Cartesian  TranslationStandardOffset=0  TranslationLengthUnit=m  TranslationStandardAxis=+Y  TranslationCartesianOffset=mParams.bodies.trunk.CG_LH  TranslationROffset=0  TranslationROffsetUnits=m  TranslationZOffset=0  TranslationZOffsetUnits=m  TranslationThetaOffset=0  TranslationThetaOffsetUnits=deg  RotationMethod=None  RotationAngleUnits=deg  RotationStandardAxis=+X  RotationAngle=90  RotationArbitraryAxis=[0 0 1]  FollAlignAxisA=+X  BaseAlignAxisA=+Y  FollAlignAxisB=+Y  BaseAlignAxisB=+Z  RotationSequenceAxes=FollowerAxes  RotationSequence=XYX  RotationSequenceAngles=[0 0 0]  RotationSequenceAnglesUnits=deg  RotationMatrix=[1 0 0; 0 1 0; 0 0 1]
  Transform CG to RH : sm_lib/Frames and Transforms/Rigid Transform  TranslationMethod=Cartesian  TranslationStandardOffset=-0  TranslationLengthUnit=m  TranslationStandardAxis=+Y  TranslationCartesianOffset=mParams.bodies.trunk.CG_RH  TranslationROffset=0  TranslationROffsetUnits=m  TranslationZOffset=0  TranslationZOffsetUnits=m  TranslationThetaOffset=0  TranslationThetaOffsetUnits=deg  RotationMethod=None  RotationAngleUnits=deg  RotationStandardAxis=+X  RotationAngle=90  RotationArbitraryAxis=[0 0 1]  FollAlignAxisA=+X  BaseAlignAxisA=+Y  FollAlignAxisB=+Y  BaseAlignAxisB=+Z  RotationSequenceAxes=FollowerAxes  RotationSequence=XYX  RotationSequenceAngles=[0 0 0]  RotationSequenceAnglesUnits=deg  RotationMatrix=[1 0 0; 0 1 0; 0 0 1]
  CG : PMIOPort  Side=Left
  Left Hip : PMIOPort  Port=2  Side=Right
  Right Hip : PMIOPort  Port=3  Side=Right
  connections:
  Solid/LConn1 -- Transform CG to RH/LConn1 -- Transform CG to LH/LConn1 -- CG/RConn1
  Left Hip/RConn1 -- Transform CG to LH/RConn1
  Right Hip/RConn1 -- Transform CG to RH/RConn1

== system nmsRR/Body and Contact Model/Vestibular System ==
  Ankle Position Right [m] : Inport
  Ankle Position Left [m] : Inport  Port=2
  "  XYZ Sensor Left Hip" : Subsystem
  "  XYZ Sensor Right Hip" : Subsystem
  Align Axis : Subsystem
  Compare To Constant : simulink/Logic and Bit Operations/Compare To Constant  relop=<=  const=1  OutDataTypeStr=boolean
  Mux : Mux  Inputs=7
  Mux1 : Mux
  R Movement direction : Subsystem
  Selector : Selector  InputPortWidth=3  IndexOptions=Index vector (dialog)  Indices=[2]  OutputSizes=1
  Stop Simulation : Stop
  Terminator : Terminator
  Terminator1 : Terminator
  To Workspace1 : ToWorkspace  VariableName=SensorBodyFrame  SampleTime=-1
      settings: Save2DSignal=2-D array (concatenate along first dimension)
  To Workspace2 : ToWorkspace  VariableName=xyzHAT  SampleTime=-1
      settings: Save2DSignal=2-D array (concatenate along first dimension)
  To Workspace3 : ToWorkspace  VariableName=HipPosR  SampleTime=-1
      settings: Save2DSignal=2-D array (concatenate along first dimension)
  To Workspace4 : ToWorkspace  VariableName=HipPosL  SampleTime=-1
      settings: Save2DSignal=2-D array (concatenate along first dimension)
  To Workspace5 : ToWorkspace  VariableName=VelocityTrunk  SampleTime=-1
      settings: Save2DSignal=2-D array (concatenate along first dimension)
  "Trunk Sensor " : Subsystem
  frame : PMIOPort  Side=Left
  Right Hip : PMIOPort  Port=2  Side=Left
  Left Hip : PMIOPort  Port=3  Side=Left
  Sensor Data (world frame) : Outport
  Sensor Data (body frame) : Outport  Port=2
  tag scope: HipL=global, HipR=global, TRK_CG=global
  wires:
  Selector/1 -> Compare To Constant/1
  Compare To Constant/1 -> Stop Simulation/1
  "Trunk Sensor "/2(Velocity Trunk [m/s]) -> To Workspace5/1, Align Axis/5(Velocity Trunk [m/s]), Mux1/2
  "Trunk Sensor "/4(Rotation Trunk [rad]) -> Mux1/4
  Ankle Position Right [m]/1 -> Align Axis/1(Ankle Position Right [m])
  "  XYZ Sensor Right Hip"/1(Hip Position [m]) -> [HipR], To Workspace3/1, R Movement direction/1(Hip Right), Align Axis/7(Hip Position Right [m])
  R Movement direction/1("R ") -> Align Axis/3("R ")
  Ankle Position Left [m]/1 -> Align Axis/2(Ankle Position Left [m])
  "Trunk Sensor "/1(Position Trunk [m]) -> [TRK_CG], Selector/1, To Workspace2/1, Align Axis/4(Position Trunk [m]), Mux1/1
  "  XYZ Sensor Left Hip"/1(Hip Position [m]) -> [HipL], To Workspace4/1, Align Axis/6(Hip Position Left [m]), R Movement direction/2(Hip Left)
  "Trunk Sensor "/3(Rotation Velocity Trunk [rad/s]) -> Mux1/3
  Align Axis/7(Lateral Trunk Rotation Velocity [rad/s] (body frame)) -> Mux/7
  Align Axis/6(Saggital Trunk Rotation Velocity [rad/s] (body frame)) -> Mux/6
  Align Axis/5(Lateral Trunk Rotation [rad] (body frame)) -> Mux/5
  Align Axis/4(Saggital Trunk Rotation [rad] (body frame)) -> Mux/4
  Align Axis/3(Trunk Velocity (body frame)) -> Mux/3
  Align Axis/2(Ankle Position Right (body frame)) -> Mux/2
  Align Axis/1(Ankle Position Left (body frame)) -> Mux/1
  Mux/1 -> To Workspace1/1, Sensor Data (body frame)/1
  Mux1/1 -> Sensor Data (world frame)/1
  "  XYZ Sensor Right Hip"/2(Hip Velocity [m/s]) -> Terminator/1
  "  XYZ Sensor Left Hip"/2(Hip Velocity [m/s]) -> Terminator1/1
  connections:
  "Trunk Sensor "/LConn1 -- frame/RConn1
  "  XYZ Sensor Left Hip"/LConn1 -- Left Hip/RConn1
  "  XYZ Sensor Right Hip"/LConn1 -- Right Hip/RConn1

== system nmsRR/Body and Contact Model/World Frame ==
  Mechanism Configuration : sm_lib/Utilities/Mechanism Configuration  UniformGravity=Constant  GravityVector=[0 -9.81 0]  GravityVectorUnits=m/s^2  GravityUnits=m/s^2  LinearizationDelta=0.001  JointModeTransitionNonlinearIterations=2
  Solver Configuration : nesl_utility/Solver Configuration  PhysicalDomain=network_engine_domain  SubClassName=solver  LeftPortType=input  RightPortType=generic  Tones=[]  Harmonics=[]  SimulateNoise=off  Profile=off  UseLocalSampling=off  EnableSwitchedLinearOptims=on  FrequencyDomain=off  UseCCode=off  RelTol=0.001  AbsTol=1e-06  MinStep=1e-09  ToWorkspace=off  RevertToSquareIcSolve=off  NumHomotopyIterations=100  PhasorMode=off  PhasorModeNumHarmonics=1  DoDC=off  ResidualTolerance=1e-9  UseLocalSolver=off  LocalSolverChoice=NE_BACKWARD_EULER_ADVANCER  LocalSolverSampleTime=.001  DoFixedCost=off  MaxNonlinIter=3  MaxModeIter=2  ComputeImpulses=off  ImpulseIterations=2  LinearAlgebra=Sparse  EquationFormulation=NE_TIME_EF  DelaysMemoryBudget=1024  AutomaticFiltering=on  FilteringTimeConstant=0.001  PartitionStorageMethod=AS_NEEDED  PartitionMemoryBudget=1024  PartitionMethod=FAST
      settings: SourceProductBaseCode=PW,SS
  World Frame : sm_lib/Frames and Transforms/World Frame
  Conn1 : PMIOPort  Side=Right
  connections:
  Solver Configuration/RConn1 -- Mechanism Configuration/RConn1 -- Conn1/RConn1 -- World Frame/RConn1

== system nmsRR/CMA Data/SS_dist1 ==
  In1 : Inport
  Trigger : TriggerPort  VariantControl=(inherit)  ZeroCross=off
  To Current Workspace4 : ToWorkspace  VariableName=SSdist  SaveFormat=Structure With Time  SampleTime=-1
      settings: MaxDataPoints=3
  wires:
  In1/1 -> To Current Workspace4/1

== system nmsRR/CMA Data/Step Counter ==
  Step2 : Inport
  Step1 : Inport  Port=2
  Constant1 : Constant  Value=0
  Constant2 : Constant  Value=0
  Constant3 : Constant  Value=0
  Constant4 : Constant  Value=-1
  Saturation Dynamic : simulink/Discontinuities/Saturation Dynamic  OutMin=[]  OutMax=[]  OutDataTypeStr=Inherit: Same as second input  OutDataType=fixdt(1, 16)  OutScaling=2^-10  DoSatur=off
  Saturation Dynamic1 : simulink/Discontinuities/Saturation Dynamic  OutMin=[]  OutMax=[]  OutDataTypeStr=Inherit: Same as second input  OutDataType=fixdt(1, 16)  OutScaling=2^-10  DoSatur=off
  Sum : Sum  Inputs=|++
  Sum1 : Sum  Inputs=++|
  Sum2 : Sum  Inputs=|++
  count steps1 : Subsystem  TreatAsAtomicUnit=on
  count steps2 : Subsystem  TreatAsAtomicUnit=on
  nStep : Outport  VectorParamsAs1DForOutWhenUnconnected=off
  wires:
  count steps1/1(nStep) -> Saturation Dynamic1/2, Sum2/2, Sum/2
  count steps2/1(nStep) -> Saturation Dynamic/2, Sum1/1, Sum/1
  Constant3/1 -> Saturation Dynamic/3
  Saturation Dynamic/1 -> count steps2/1(nStep-1)
  Constant1/1 -> Sum1/2
  Sum1/1 -> Saturation Dynamic1/1
  Constant2/1 -> Saturation Dynamic1/3
  Saturation Dynamic1/1 -> count steps1/1(nStep-1)
  Constant4/1 -> Sum2/1
  Sum2/1 -> Saturation Dynamic/1
  Step2/1 -> count steps2/Trigger
  Sum/1 -> nStep/1
  Step1/1 -> count steps1/Trigger
